simulink model "StartFromStrach"  (Simulink 8.8)
settings: Solver=FixedStepDiscrete  StartTime=0.0  StopTime=CONFIG.SIMULATION_TIME  FixedStep=CONFIG.Ts  RelTol=1e-3  EnableMultiTasking=on
InitFcn:
  | cd(fileparts(which(bdroot)));
  | initStartFromScratch;
undefined symbols (not defined in the file or in its folder): CONFIG, ConstraintsFeetMatrix, gain, reg, ROBOT_DOF, sat, sm, upperBoundFeetConstraints, WBT_robotName
libraries: WBToolboxLibrary x47
settings Model: SuppressorTable=22 serialization::archive 11 0 3 0 0 0 11 0  Creator=marie  LastModifiedBy=marie
settings DataIOCC: LimitDataPoints=off  SaveFormat=Dataset  SignalLoggingSaveFormat=Dataset
settings OptimizationCC: LifeSpan=auto
settings DebuggingCC: UnderspecifiedInitializationDetection=Simplified  MergeDetectMultiDrivingBlocksExec=error  FcnCallInpInsideContextMsg=error  StateNameClashWarn=none  SFUnexpectedBacktrackingDiag=error  SFNoUnconditionalDefaultTransitionDiag=error  SFExecutionAtInitializationDiag=warning
settings HardwareCC: ProdBitPerPointer=64  ProdBitPerSizeT=64  ProdBitPerPtrDiffT=64  ProdLargestAtomicFloat=Float  ProdIntDivRoundTo=Zero  ProdEndianess=LittleEndian  ProdWordSize=64  ProdHWDeviceType=Intel->x86-64 (Windows64)
settings ModelReferenceCC: PropagateSignalLabelsOutOfModel=on
settings GRTTargetCC: TargetLangStandard=C99 (ISO)  GeneratePreprocessorConditionals=Use local settings  CombineOutputUpdateFcns=on  GRTInterface=off
settings ConfigComp: CovMetricSettings=dwe  CovHtmlReporting=off  CovSaveCumulativeToWorkspaceVar=off  CovSaveSingleToWorkspaceVar=off  CovExternalEMLEnable=on

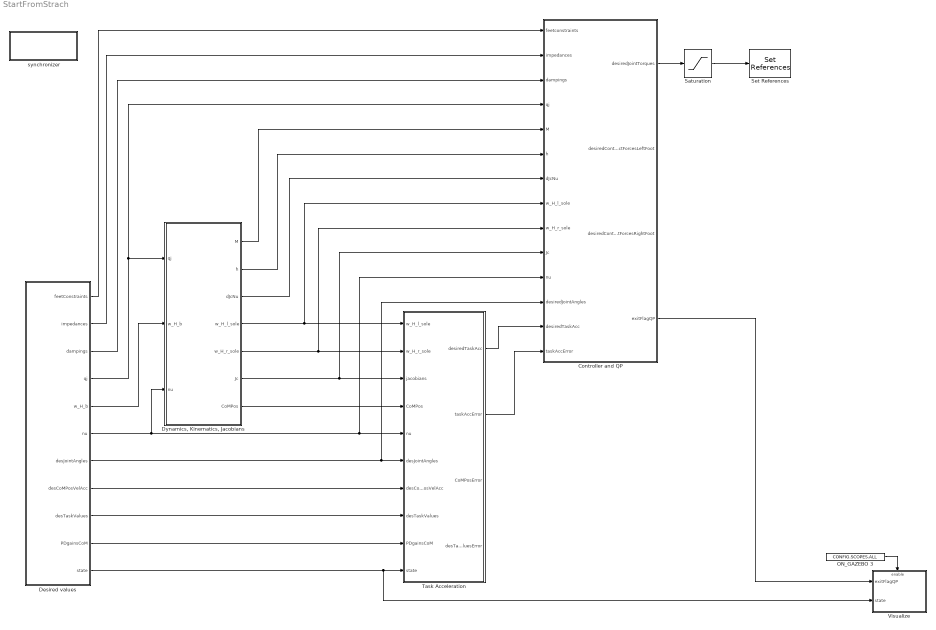
== system StartFromStrach ==
  Controller and QP : Subsystem
  Desired values : Subsystem
  "Dynamics, Kinematics, Jacobians" : Subsystem
  ON_GAZEBO 3 : Constant  Value=CONFIG.SCOPES.ALL
  Saturation : Saturate  UpperLimit=sat.torque  LowerLimit=-sat.torque
  Set References : WBToolboxLibrary/wholeBodyActuators/Set References  controlType=Torque  fullOrSubControl=Full  controlledJoints=''  robotName=WBT_robotName  localName=WBT_modelName  wbiFile=WBT_wbiFilename  wbiList=WBT_wbiList
  Task Acceleration : Subsystem
  Visualize : Subsystem
  synchronizer : Subsystem
      mask Display: disp('SYNCHRONIZER')
  wires:
  Desired values/5(w_H_b) -> "Dynamics, Kinematics, Jacobians"/2(w_H_b)
  Desired values/4(qj) -> "Dynamics, Kinematics, Jacobians"/1(qj), Controller and QP/4(qj)
  "Dynamics, Kinematics, Jacobians"/7(CoMPos) -> Task Acceleration/4(CoMPos)
  Desired values/8(desCoMPosVelAcc) -> Task Acceleration/7(desCoMPosVelAcc)
  Desired values/6(nu) -> Controller and QP/11(nu), Task Acceleration/5(nu), "Dynamics, Kinematics, Jacobians"/3(nu)
  "Dynamics, Kinematics, Jacobians"/6(Jc) -> Controller and QP/10(Jc), Task Acceleration/3(jacobians)
  Desired values/7(desJointAngles) -> Task Acceleration/6(desJointAngles), Controller and QP/12(desiredJointAngles)
  Desired values/9(desTaskValues) -> Task Acceleration/8(desTaskValues)
  Desired values/10(PDgainsCoM) -> Task Acceleration/9(PDgainsCoM)
  "Dynamics, Kinematics, Jacobians"/5(w_H_r_sole) -> Controller and QP/9(w_H_r_sole), Task Acceleration/2(w_H_r_sole)
  "Dynamics, Kinematics, Jacobians"/4(w_H_l_sole) -> Controller and QP/8(w_H_l_sole), Task Acceleration/1(w_H_l_sole)
  Desired values/2(impedances) -> Controller and QP/2(impedances)
  Desired values/1(feetConstraints) -> Controller and QP/1(feetconstraints)
  "Dynamics, Kinematics, Jacobians"/1(M) -> Controller and QP/5(M)
  "Dynamics, Kinematics, Jacobians"/2(h) -> Controller and QP/6(h)
  "Dynamics, Kinematics, Jacobians"/3(dJcNu) -> Controller and QP/7(dJcNu)
  Task Acceleration/1(desiredTaskAcc) -> Controller and QP/13(desiredTaskAcc)
  Task Acceleration/2(taskAccError) -> Controller and QP/14(taskAccError)
  Desired values/3(dampings) -> Controller and QP/3(dampings)
  Controller and QP/1(desiredJointTorques) -> Saturation/1
  Saturation/1 -> Set References/1
  ON_GAZEBO 3/1 -> Visualize/Enable
  Desired values/11(state) -> Visualize/2(state), Task Acceleration/10(state)
  Controller and QP/4(exitFlagQP) -> Visualize/1(exitFlagQP)

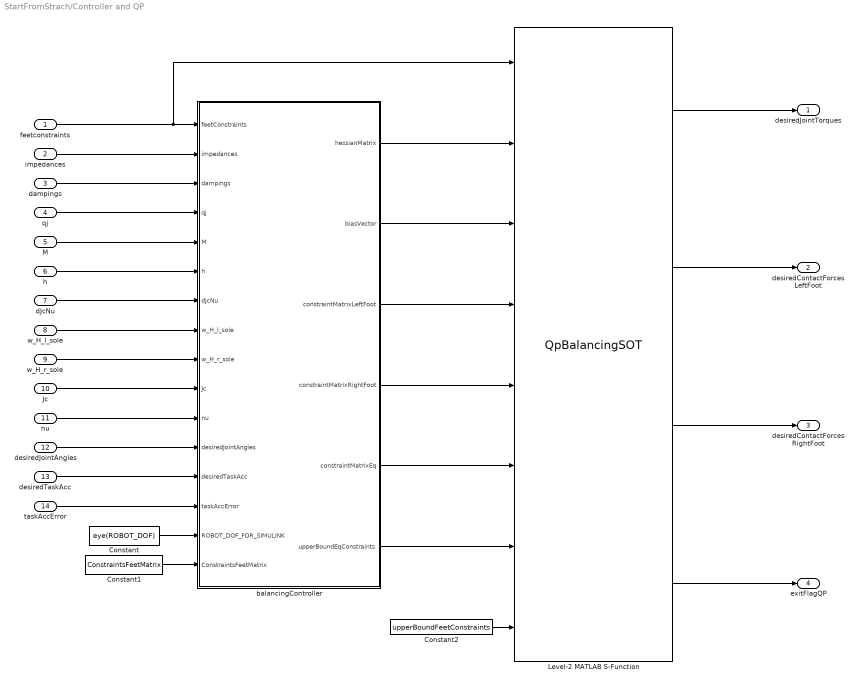
== system StartFromStrach/Controller and QP ==
  feetconstraints : Inport
  impedances : Inport  Port=2
  dampings : Inport  Port=3
  qj : Inport  Port=4
  M : Inport  Port=5
  h : Inport  Port=6
  dJcNu : Inport  Port=7
  w_H_l_sole : Inport  Port=8
  w_H_r_sole : Inport  Port=9
  Jc : Inport  Port=10
  nu : Inport  Port=11
  desiredJointAngles : Inport  Port=12
  desiredTaskAcc : Inport  Port=13
  taskAccError : Inport  Port=14
  Constant : Constant  Value=eye(ROBOT_DOF)
  Constant1 : Constant  Value=ConstraintsFeetMatrix
  Constant2 : Constant  Value=upperBoundFeetConstraints
  Level-2 MATLAB S-Function : M-S-Function  FunctionName=QpBalancingSOT  Parameters=ROBOT_DOF,sat.torqueDot,CONFIG.Ts,CONFIG.QP.USE_CONTINUITY_CONSTRAINTS,CONFIG.QP.USE_STRICT_TASK_PRIORITIES, reg.HessianQP  mask{robotDofs=ROBOT_DOF, tauDotMax=sat.torqueDot, Ts=CONFIG.Ts}
      mask prompts: robotDofs "Robt degrees of freedom"; tauDotMax "Maximum derivative of torques"; Ts "Controller period"
      mask Display: disp('QP')
  balancingController : MATLAB Function  TreatAsAtomicUnit=on
  desiredJointTorques : Outport
  desiredContactForcesLeftFoot : Outport  Port=2
  desiredContactForcesRightFoot : Outport  Port=3
  exitFlagQP : Outport  Port=4
  wires:
  balancingController/1(hessianMatrix) -> Level-2 MATLAB S-Function/2
  feetconstraints/1 -> Level-2 MATLAB S-Function/1, balancingController/1(feetConstraints)
  qj/1 -> balancingController/4(qj)
  impedances/1 -> balancingController/2(impedances)
  M/1 -> balancingController/5(M)
  h/1 -> balancingController/6(h)
  dJcNu/1 -> balancingController/7(dJcNu)
  w_H_l_sole/1 -> balancingController/8(w_H_l_sole)
  w_H_r_sole/1 -> balancingController/9(w_H_r_sole)
  Jc/1 -> balancingController/10(Jc)
  nu/1 -> balancingController/11(nu)
  desiredJointAngles/1 -> balancingController/12(desiredJointAngles)
  desiredTaskAcc/1 -> balancingController/13(desiredTaskAcc)
  taskAccError/1 -> balancingController/14(taskAccError)
  Constant/1 -> balancingController/15(ROBOT_DOF_FOR_SIMULINK)
  Constant1/1 -> balancingController/16(ConstraintsFeetMatrix)
  dampings/1 -> balancingController/3(dampings)
  balancingController/2(biasVector) -> Level-2 MATLAB S-Function/3
  balancingController/3(constraintMatrixLeftFoot) -> Level-2 MATLAB S-Function/4
  balancingController/4(constraintMatrixRightFoot) -> Level-2 MATLAB S-Function/5
  balancingController/5(constraintMatrixEq) -> Level-2 MATLAB S-Function/6
  balancingController/6(upperBoundEqConstraints) -> Level-2 MATLAB S-Function/7
  Constant2/1 -> Level-2 MATLAB S-Function/8
  Level-2 MATLAB S-Function/1 -> desiredJointTorques/1
  Level-2 MATLAB S-Function/2 -> desiredContactForcesLeftFoot/1
  Level-2 MATLAB S-Function/3 -> desiredContactForcesRightFoot/1
  Level-2 MATLAB S-Function/4 -> exitFlagQP/1

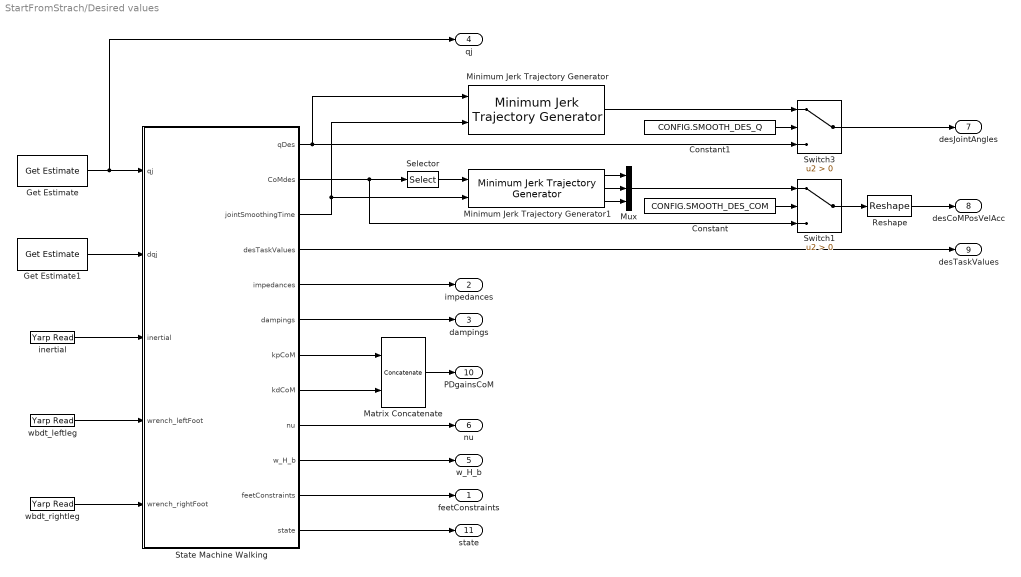
== system StartFromStrach/Desired values ==
  Constant : Constant  Value=CONFIG.SMOOTH_DES_COM
  Constant1 : Constant  Value=CONFIG.SMOOTH_DES_Q
  Get Estimate : WBToolboxLibrary/wholeBodyStates/Get Estimate  estimateType=Joints Position  robotName=WBT_robotName  localName=WBT_modelName  wbiFile=WBT_wbiFilename  wbiList=WBT_wbiList
  Get Estimate1 : WBToolboxLibrary/wholeBodyStates/Get Estimate  estimateType=Joints Velocity  robotName=WBT_robotName  localName=WBT_modelName  wbiFile=WBT_wbiFilename  wbiList=WBT_wbiList
  Matrix Concatenate : Concatenate  Mode=Multidimensional array  ConcatenateDimension=2
  Minimum Jerk Trajectory Generator : WBToolboxLibrary/Utilities/Minimum Jerk Trajectory Generator  externalSettlingTime=on  settlingTime=3  sampleTime=CONFIG.Ts  resetOnSettlingTime=off  firstDerivatives=off  secondDerivatives=off  explicitInitialValue=off
  Minimum Jerk Trajectory Generator1 : WBToolboxLibrary/Utilities/Minimum Jerk Trajectory Generator  externalSettlingTime=on  settlingTime=3  sampleTime=CONFIG.Ts  resetOnSettlingTime=off  firstDerivatives=on  secondDerivatives=on  explicitInitialValue=off
  Mux : Mux  Inputs=3
  Reshape : Reshape  OutputDimensionality=Customize  OutputDimensions=[3,3]
  Selector : Selector  InputPortWidth=9  IndexOptions=Index vector (dialog)  Indices=[1 2 3]  OutputSizes=1
  State Machine Walking : Subsystem
  Switch1 : Switch  Criteria=u2 > Threshold
  Switch3 : Switch  Criteria=u2 > Threshold
  inertial : WBToolboxLibrary/Utilities/Yarp Read  portName=PORTS.IMU  signalSize=12  blocking=off  timestamp=off  autoconnect=on  errorOnConnection=on
  wbdt_leftleg : WBToolboxLibrary/Utilities/Yarp Read  portName=PORTS.WBDT_LEFTLEG_EE  signalSize=6  blocking=off  timestamp=off  autoconnect=on  errorOnConnection=off
  wbdt_rightleg : WBToolboxLibrary/Utilities/Yarp Read  portName=PORTS.WBDT_RIGHTLEG_EE  signalSize=6  blocking=off  timestamp=off  autoconnect=on  errorOnConnection=off
  feetConstraints : Outport
  impedances : Outport  Port=2
  dampings : Outport  Port=3
  qj : Outport  Port=4
  w_H_b : Outport  Port=5
  nu : Outport  Port=6
  desJointAngles : Outport  Port=7
  desCoMPosVelAcc : Outport  Port=8
  desTaskValues : Outport  Port=9
  PDgainsCoM : Outport  Port=10
  state : Outport  Port=11
  wires:
  Minimum Jerk Trajectory Generator/1 -> Switch3/1
  Constant/1 -> Switch1/2
  Constant1/1 -> Switch3/2
  Minimum Jerk Trajectory Generator1/3 -> Mux/3
  Minimum Jerk Trajectory Generator1/2 -> Mux/2
  State Machine Walking/8(kdCoM) -> Matrix Concatenate/2
  Matrix Concatenate/1 -> PDgainsCoM/1
  State Machine Walking/10(w_H_b) -> w_H_b/1
  State Machine Walking/12(state) -> state/1
  Mux/1 -> Switch1/1
  Minimum Jerk Trajectory Generator1/1 -> Mux/1
  State Machine Walking/5(impedances) -> impedances/1
  Selector/1 -> Minimum Jerk Trajectory Generator1/1
  State Machine Walking/3(jointSmoothingTime) -> Minimum Jerk Trajectory Generator/2, Minimum Jerk Trajectory Generator1/2
  Switch1/1 -> Reshape/1
  Switch3/1 -> desJointAngles/1
  State Machine Walking/2(CoMdes) -> Switch1/3, Selector/1
  State Machine Walking/4(desTaskValues) -> desTaskValues/1
  State Machine Walking/11(feetConstraints) -> feetConstraints/1
  State Machine Walking/1(qDes) -> Minimum Jerk Trajectory Generator/1, Switch3/3
  State Machine Walking/9(nu) -> nu/1
  State Machine Walking/7(kpCoM) -> Matrix Concatenate/1
  Reshape/1 -> desCoMPosVelAcc/1
  inertial/1 -> State Machine Walking/3(inertial)
  Get Estimate/1 -> qj/1, State Machine Walking/1(qj)
  Get Estimate1/1 -> State Machine Walking/2(dqj)
  wbdt_leftleg/1 -> State Machine Walking/4(wrench_leftFoot)
  wbdt_rightleg/1 -> State Machine Walking/5(wrench_rightFoot)
  State Machine Walking/6(dampings) -> dampings/1

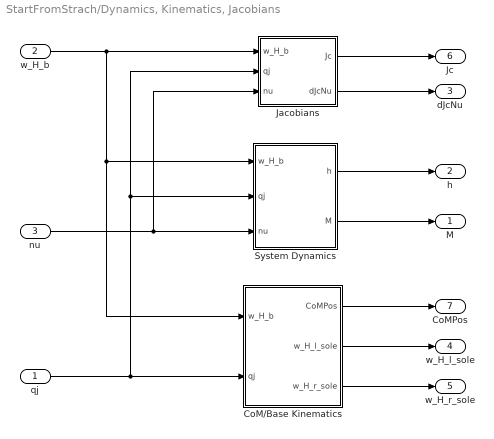
== system StartFromStrach/Dynamics, Kinematics, Jacobians ==
  qj : Inport
  w_H_b : Inport  Port=2
  nu : Inport  Port=3
  CoM/Base Kinematics : Subsystem
  Jacobians : Subsystem
  System Dynamics : Subsystem
  M : Outport
  h : Outport  Port=2
  dJcNu : Outport  Port=3
  w_H_l_sole : Outport  Port=4
  w_H_r_sole : Outport  Port=5
  Jc : Outport  Port=6
  CoMPos : Outport  Port=7
  wires:
  qj/1 -> Jacobians/2(qj), System Dynamics/2(qj), CoM/Base Kinematics/2(qj)
  w_H_b/1 -> CoM/Base Kinematics/1(w_H_b), System Dynamics/1(w_H_b), Jacobians/1(w_H_b)
  CoM/Base Kinematics/1(CoMPos) -> CoMPos/1
  nu/1 -> Jacobians/3(nu), System Dynamics/3(nu)
  Jacobians/1(Jc) -> Jc/1
  Jacobians/2(dJcNu) -> dJcNu/1
  System Dynamics/2(M) -> M/1
  System Dynamics/1(h) -> h/1
  CoM/Base Kinematics/2(w_H_l_sole) -> w_H_l_sole/1
  CoM/Base Kinematics/3(w_H_r_sole) -> w_H_r_sole/1

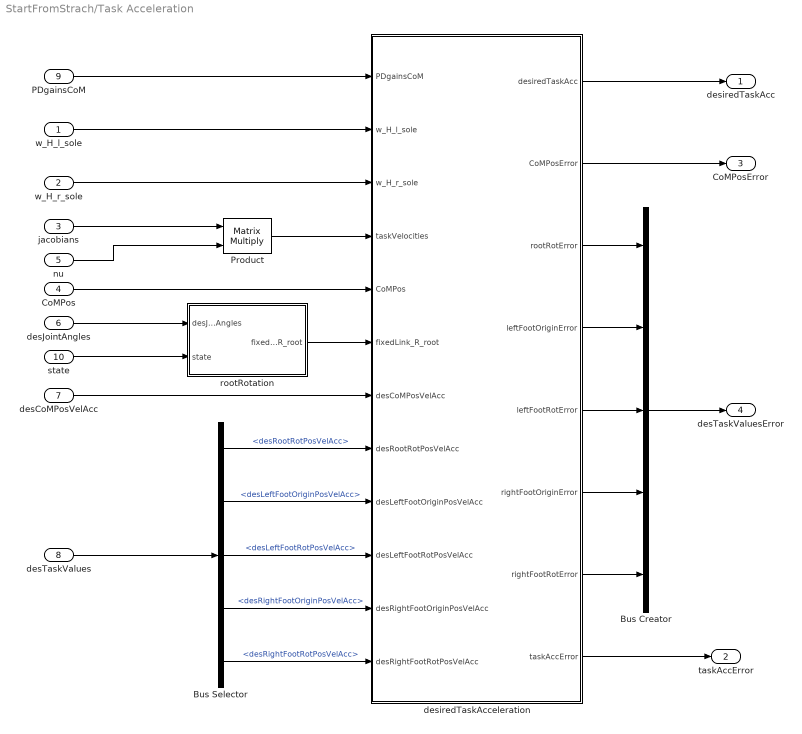
== system StartFromStrach/Task Acceleration ==
  w_H_l_sole : Inport
  w_H_r_sole : Inport  Port=2
  jacobians : Inport  Port=3
  CoMPos : Inport  Port=4
  nu : Inport  Port=5
  desJointAngles : Inport  Port=6
  desCoMPosVelAcc : Inport  Port=7
  desTaskValues : Inport  Port=8
  PDgainsCoM : Inport  Port=9
  state : Inport  Port=10
  Bus Creator : BusCreator  Inputs='rootRotError','leftFootOriginError','leftFootRotError','rightFootOriginError','rightFootRotError'
  Bus Selector : BusSelector  OutputSignals=desRootRotPosVelAcc,desLeftFootOriginPosVelAcc,desLeftFootRotPosVelAcc,desRightFootOriginPosVelAcc,desRightFootRotPosVelAcc
  Product : Product  Multiplication=Matrix(*)
  desiredTaskAcceleration : MATLAB Function  TreatAsAtomicUnit=on
  rootRotation : Subsystem
  desiredTaskAcc : Outport
  taskAccError : Outport  Port=2
  CoMPosError : Outport  Port=3
  desTaskValuesError : Outport  Port=4
  wires:
  state/1 -> rootRotation/2(state)
  Bus Selector/1 -> desiredTaskAcceleration/8(desRootRotPosVelAcc)  "<desRootRotPosVelAcc>"
  Bus Selector/2 -> desiredTaskAcceleration/9(desLeftFootOriginPosVelAcc)  "<desLeftFootOriginPosVelAcc>"
  desJointAngles/1 -> rootRotation/1(desJointAngles)
  Bus Selector/3 -> desiredTaskAcceleration/10(desLeftFootRotPosVelAcc)  "<desLeftFootRotPosVelAcc>"
  Bus Selector/4 -> desiredTaskAcceleration/11(desRightFootOriginPosVelAcc)  "<desRightFootOriginPosVelAcc>"
  desTaskValues/1 -> Bus Selector/1
  rootRotation/1(fixedLink_R_root) -> desiredTaskAcceleration/6(fixedLink_R_root)
  Bus Selector/5 -> desiredTaskAcceleration/12(desRightFootRotPosVelAcc)  "<desRightFootRotPosVelAcc>"
  PDgainsCoM/1 -> desiredTaskAcceleration/1(PDgainsCoM)
  jacobians/1 -> Product/1
  nu/1 -> Product/2
  CoMPos/1 -> desiredTaskAcceleration/5(CoMPos)
  desCoMPosVelAcc/1 -> desiredTaskAcceleration/7(desCoMPosVelAcc)
  Product/1 -> desiredTaskAcceleration/4(taskVelocities)
  desiredTaskAcceleration/3(rootRotError) -> Bus Creator/1
  desiredTaskAcceleration/4(leftFootOriginError) -> Bus Creator/2
  desiredTaskAcceleration/5(leftFootRotError) -> Bus Creator/3
  desiredTaskAcceleration/6(rightFootOriginError) -> Bus Creator/4
  desiredTaskAcceleration/7(rightFootRotError) -> Bus Creator/5
  desiredTaskAcceleration/1(desiredTaskAcc) -> desiredTaskAcc/1
  desiredTaskAcceleration/2(CoMPosError) -> CoMPosError/1
  Bus Creator/1 -> desTaskValuesError/1
  desiredTaskAcceleration/8(taskAccError) -> taskAccError/1
  w_H_r_sole/1 -> desiredTaskAcceleration/3(w_H_r_sole)
  w_H_l_sole/1 -> desiredTaskAcceleration/2(w_H_l_sole)

== system StartFromStrach/Visualize ==
  exitFlagQP : Inport
  state : Inport  Port=2
  Enable : EnablePort
  ON_GAZEBO 4 : Constant  Value=CONFIG.SCOPES.QP
  Visualize eventual QP failures : Subsystem
  wires:
  state/1 -> Visualize eventual QP failures/2(state)
  ON_GAZEBO 4/1 -> Visualize eventual QP failures/Enable
  exitFlagQP/1 -> Visualize eventual QP failures/1(exitFlagQP)

== system StartFromStrach/synchronizer ==
  GAZEBO_SYNCHRONIZER : Subsystem
  Logical Operator : Logic  Operator=NOT  AllPortsSameDT=off  OutDataTypeStr=boolean
  "ON_GAZEBO " : Constant  Value=CONFIG.ON_GAZEBO
  REAL_TIME_SYNC : Subsystem
  wires:
  Logical Operator/1 -> REAL_TIME_SYNC/Enable
  "ON_GAZEBO "/1 -> GAZEBO_SYNCHRONIZER/Enable, Logical Operator/1

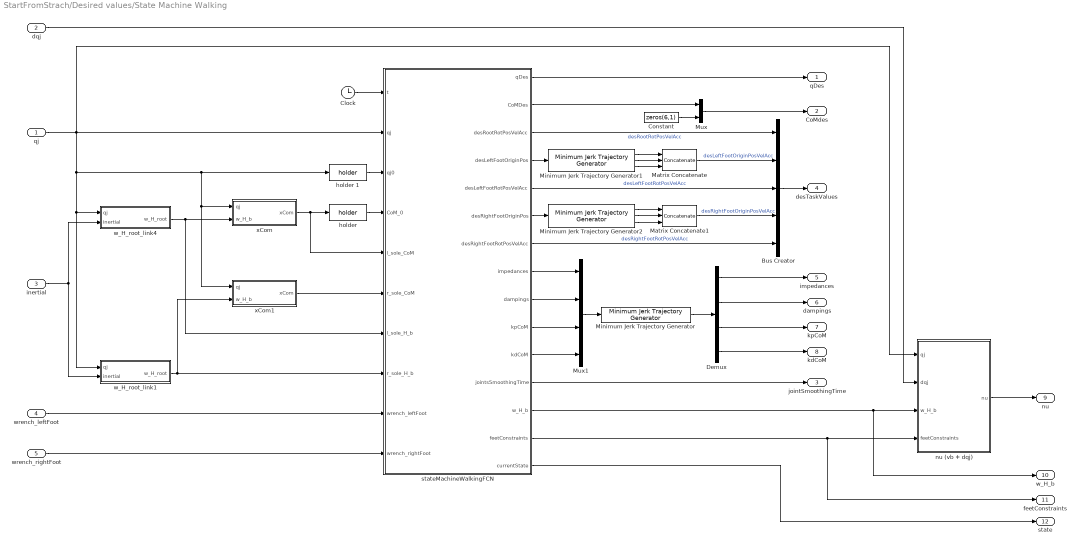
== system StartFromStrach/Desired values/State Machine Walking ==
  qj : Inport
  dqj : Inport  Port=2
  inertial : Inport  Port=3
  wrench_leftFoot : Inport  Port=4
  wrench_rightFoot : Inport  Port=5
  Bus Creator : BusCreator  Inputs='desRootRotPosVelAcc','desLeftFootOriginPosVelAcc','desLeftFootRotPosVelAcc','desRightFootOriginPosVelAcc','desRightFootRotPosVelAcc'
  Clock : Clock
  Constant : Constant  Value=zeros(6,1)
  Demux : Demux  Outputs=[ROBOT_DOF, ROBOT_DOF, 3, 3]
  Matrix Concatenate : Concatenate  NumInputs=3  Mode=Multidimensional array  ConcatenateDimension=2
  Matrix Concatenate1 : Concatenate  NumInputs=3  Mode=Multidimensional array  ConcatenateDimension=2
  Minimum Jerk Trajectory Generator : WBToolboxLibrary/Utilities/Minimum Jerk Trajectory Generator  externalSettlingTime=off  settlingTime=gain.SmoothingTimeGainScheduling  sampleTime=CONFIG.Ts  resetOnSettlingTime=off  firstDerivatives=off  secondDerivatives=off  explicitInitialValue=off
  Minimum Jerk Trajectory Generator1 : WBToolboxLibrary/Utilities/Minimum Jerk Trajectory Generator  externalSettlingTime=off  settlingTime=gain.SmoothingTimeGainScheduling  sampleTime=CONFIG.Ts  resetOnSettlingTime=off  firstDerivatives=on  secondDerivatives=on  explicitInitialValue=off
  Minimum Jerk Trajectory Generator2 : WBToolboxLibrary/Utilities/Minimum Jerk Trajectory Generator  externalSettlingTime=off  settlingTime=gain.SmoothingTimeGainScheduling  sampleTime=CONFIG.Ts  resetOnSettlingTime=off  firstDerivatives=on  secondDerivatives=on  explicitInitialValue=off
  Mux : Mux  Inputs=2
  Mux1 : Mux
  "holder " : WBToolboxLibrary/Utilities/holder 
  holder 1 : WBToolboxLibrary/Utilities/holder 
  nu (vb + dqj) : Subsystem
  stateMachineWalkingFCN : MATLAB Function  TreatAsAtomicUnit=on
  w_H_root_link1 : Subsystem  mask{link_name='r_sole'}
      mask prompts: link_name "link name"
      mask help:
      | This block evaluates the homogeneous transformation between the world and the root link, i.e. ^wH_b. It assumes that the link specified by the variable 'link_name' has a constant position
      | w.r.t. an inertial frame, but it can rotate arbitrarily. This rotation is retrived from the IMU sensor.
      mask Display:
      | str = strrep(link_name, '_','\_');
      | port_label('output',1,['{}^{',str '}H_{root}'],'texmode','on')
      | clear str;
      | 
      | port_label('input',1,'q_j','texmode','on')
      | 
      | port_label('input',2,'inertial','texmode','on')
  w_H_root_link4 : Subsystem  mask{link_name='l_sole'}
      mask prompts: link_name "link name"
      mask help:
      | This block evaluates the homogeneous transformation between the world and the root link, i.e. ^wH_b. It assumes that the link specified by the variable 'link_name' has a constant position
      | w.r.t. an inertial frame, but it can rotate arbitrarily. This rotation is retrived from the IMU sensor.
      mask Display:
      | str = strrep(link_name, '_','\_');
      | port_label('output',1,['{}^{',str '}H_{root}'],'texmode','on')
      | clear str;
      | 
      | port_label('input',1,'q_j','texmode','on')
      | 
      | port_label('input',2,'inertial','texmode','on')
  xCom : Subsystem
  xCom1 : Subsystem
  qDes : Outport
  CoMdes : Outport  Port=2
  jointSmoothingTime : Outport  Port=3
  desTaskValues : Outport  Port=4
  impedances : Outport  Port=5
  dampings : Outport  Port=6
  kpCoM : Outport  Port=7
  kdCoM : Outport  Port=8
  nu : Outport  Port=9
  w_H_b : Outport  Port=10
  feetConstraints : Outport  Port=11
  state : Outport  Port=12
  wires:
  Clock/1 -> stateMachineWalkingFCN/1(t)
  stateMachineWalkingFCN/8(impedances) -> Mux1/1
  stateMachineWalkingFCN/11(kdCoM) -> Mux1/4
  stateMachineWalkingFCN/7(desRightFootRotPosVelAcc) -> Bus Creator/5  "desRightFootRotPosVelAcc"
  Bus Creator/1 -> desTaskValues/1
  wrench_rightFoot/1 -> stateMachineWalkingFCN/10(wrench_rightFoot)
  stateMachineWalkingFCN/10(kpCoM) -> Mux1/3
  stateMachineWalkingFCN/13(w_H_b) -> w_H_b/1, nu (vb + dqj)/3(w_H_b)
  wrench_leftFoot/1 -> stateMachineWalkingFCN/9(wrench_leftFoot)
  Mux1/1 -> Minimum Jerk Trajectory Generator/1
  qj/1 -> nu (vb + dqj)/1(qj), w_H_root_link1/1(qj), w_H_root_link4/1(qj), xCom1/1(qj), xCom/1(qj), holder 1/1, stateMachineWalkingFCN/2(qj)
  nu (vb + dqj)/1(nu) -> nu/1
  holder 1/1 -> stateMachineWalkingFCN/3(qj0)
  xCom1/1(xCom) -> stateMachineWalkingFCN/6(r_sole_CoM)
  "holder "/1 -> stateMachineWalkingFCN/4(CoM_0)
  w_H_root_link4/1(w_H_root) -> stateMachineWalkingFCN/7(l_sole_H_b), xCom/2(w_H_b)
  inertial/1 -> w_H_root_link4/2(inertial), w_H_root_link1/2(inertial)
  xCom/1(xCom) -> "holder "/1, stateMachineWalkingFCN/5(l_sole_CoM)
  Minimum Jerk Trajectory Generator/1 -> Demux/1
  stateMachineWalkingFCN/14(feetConstraints) -> nu (vb + dqj)/4(feetConstraints), feetConstraints/1
  dqj/1 -> nu (vb + dqj)/2(dqj)
  stateMachineWalkingFCN/2(CoMDes) -> Mux/1
  w_H_root_link1/1(w_H_root) -> xCom1/2(w_H_b), stateMachineWalkingFCN/8(r_sole_H_b)
  Demux/1 -> impedances/1
  stateMachineWalkingFCN/12(jointsSmoothingTime) -> jointSmoothingTime/1
  stateMachineWalkingFCN/15(currentState) -> state/1
  stateMachineWalkingFCN/1(qDes) -> qDes/1
  Demux/3 -> kpCoM/1
  Minimum Jerk Trajectory Generator1/1 -> Matrix Concatenate/1
  Minimum Jerk Trajectory Generator1/2 -> Matrix Concatenate/2
  Minimum Jerk Trajectory Generator1/3 -> Matrix Concatenate/3
  Matrix Concatenate/1 -> Bus Creator/2  "desLeftFootOriginPosVelAcc"
  stateMachineWalkingFCN/4(desLeftFootOriginPos) -> Minimum Jerk Trajectory Generator1/1
  Minimum Jerk Trajectory Generator2/1 -> Matrix Concatenate1/1
  Minimum Jerk Trajectory Generator2/2 -> Matrix Concatenate1/2
  Minimum Jerk Trajectory Generator2/3 -> Matrix Concatenate1/3
  stateMachineWalkingFCN/6(desRightFootOriginPos) -> Minimum Jerk Trajectory Generator2/1
  Matrix Concatenate1/1 -> Bus Creator/4  "desRightFootOriginPosVelAcc"
  stateMachineWalkingFCN/3(desRootRotPosVelAcc) -> Bus Creator/1  "desRootRotPosVelAcc"
  stateMachineWalkingFCN/5(desLeftFootRotPosVelAcc) -> Bus Creator/3  "desLeftFootRotPosVelAcc"
  Demux/4 -> kdCoM/1
  Constant/1 -> Mux/2
  Mux/1 -> CoMdes/1
  stateMachineWalkingFCN/9(dampings) -> Mux1/2
  Demux/2 -> dampings/1

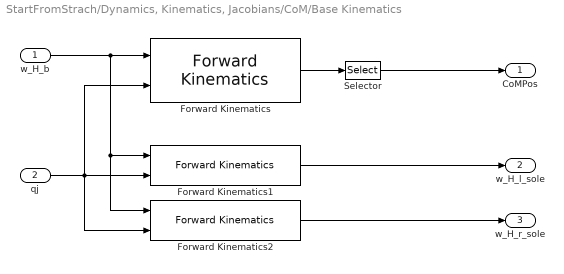
== system StartFromStrach/Dynamics, Kinematics, Jacobians/CoM/Base Kinematics ==
  w_H_b : Inport
  qj : Inport  Port=2
  Forward Kinematics : WBToolboxLibrary/wholeBodyModel/Kinematics/Forward Kinematics  frameName='com'  robotName=WBT_robotName  localName=WBT_modelName  wbiFile=WBT_wbiFilename  wbiList=WBT_wbiList
  Forward Kinematics1 : WBToolboxLibrary/wholeBodyModel/Kinematics/Forward Kinematics  frameName='l_sole'  robotName=WBT_robotName  localName=WBT_modelName  wbiFile=WBT_wbiFilename  wbiList=WBT_wbiList
  Forward Kinematics2 : WBToolboxLibrary/wholeBodyModel/Kinematics/Forward Kinematics  frameName='r_sole'  robotName=WBT_robotName  localName=WBT_modelName  wbiFile=WBT_wbiFilename  wbiList=WBT_wbiList
  Selector : Selector  NumberOfDimensions=2  InputPortWidth=6+ROBOT_DOF  IndexOptions=Index vector (dialog),Index vector (dialog)  Indices=[1:3],[4]  OutputSizes=1,1
  CoMPos : Outport
  w_H_l_sole : Outport  Port=2
  w_H_r_sole : Outport  Port=3
  wires:
  Selector/1 -> CoMPos/1
  qj/1 -> Forward Kinematics1/2, Forward Kinematics2/2, Forward Kinematics/2
  Forward Kinematics/1 -> Selector/1
  w_H_b/1 -> Forward Kinematics1/1, Forward Kinematics2/1, Forward Kinematics/1
  Forward Kinematics2/1 -> w_H_r_sole/1
  Forward Kinematics1/1 -> w_H_l_sole/1

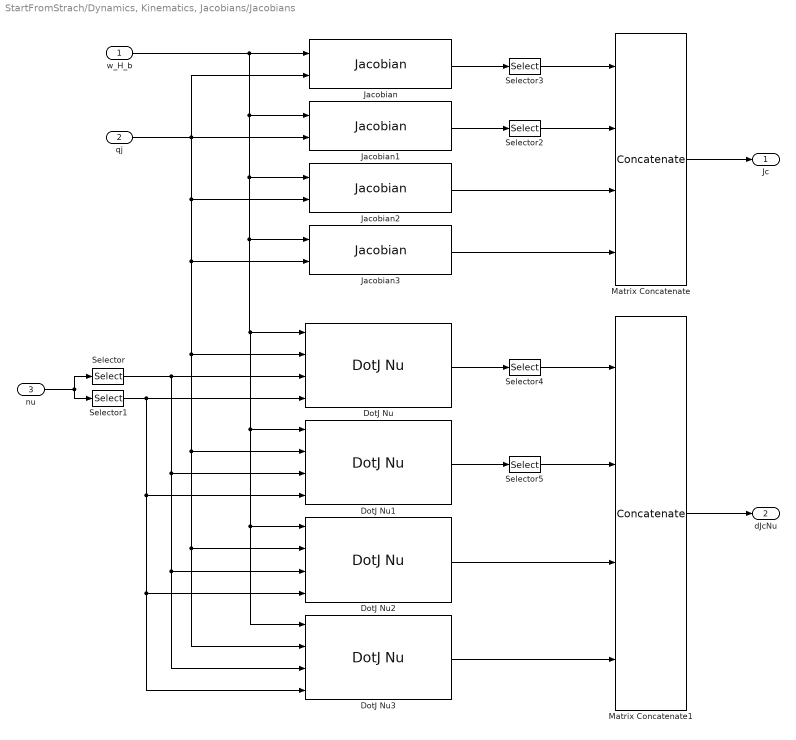
== system StartFromStrach/Dynamics, Kinematics, Jacobians/Jacobians ==
  w_H_b : Inport
  qj : Inport  Port=2
  nu : Inport  Port=3
  DotJ Nu : WBToolboxLibrary/wholeBodyModel/Jacobians/DotJ Nu  frameName='com'  robotName=WBT_robotName  localName=WBT_modelName  wbiFile=WBT_wbiFilename  wbiList=WBT_wbiList
  DotJ Nu1 : WBToolboxLibrary/wholeBodyModel/Jacobians/DotJ Nu  frameName='root_link'  robotName=WBT_robotName  localName=WBT_modelName  wbiFile=WBT_wbiFilename  wbiList=WBT_wbiList
  DotJ Nu2 : WBToolboxLibrary/wholeBodyModel/Jacobians/DotJ Nu  frameName='l_sole'  robotName=WBT_robotName  localName=WBT_modelName  wbiFile=WBT_wbiFilename  wbiList=WBT_wbiList
  DotJ Nu3 : WBToolboxLibrary/wholeBodyModel/Jacobians/DotJ Nu  frameName='r_sole'  robotName=WBT_robotName  localName=WBT_modelName  wbiFile=WBT_wbiFilename  wbiList=WBT_wbiList
  Jacobian : WBToolboxLibrary/wholeBodyModel/Jacobians/Jacobian  frameName='com'  robotName=WBT_robotName  localName=WBT_modelName  wbiFile=WBT_wbiFilename  wbiList=WBT_wbiList
  Jacobian1 : WBToolboxLibrary/wholeBodyModel/Jacobians/Jacobian  frameName='root_link'  robotName=WBT_robotName  localName=WBT_modelName  wbiFile=WBT_wbiFilename  wbiList=WBT_wbiList
  Jacobian2 : WBToolboxLibrary/wholeBodyModel/Jacobians/Jacobian  frameName='l_sole'  robotName=WBT_robotName  localName=WBT_modelName  wbiFile=WBT_wbiFilename  wbiList=WBT_wbiList
  Jacobian3 : WBToolboxLibrary/wholeBodyModel/Jacobians/Jacobian  frameName='r_sole'  robotName=WBT_robotName  localName=WBT_modelName  wbiFile=WBT_wbiFilename  wbiList=WBT_wbiList
  Matrix Concatenate : Concatenate  NumInputs=4  Mode=Multidimensional array
  Matrix Concatenate1 : Concatenate  NumInputs=4  Mode=Multidimensional array
  Selector : Selector  InputPortWidth=6+ROBOT_DOF  IndexOptions=Index vector (dialog)  Indices=[1:6]  OutputSizes=1
  Selector1 : Selector  InputPortWidth=6+ROBOT_DOF  IndexOptions=Index vector (dialog)  Indices=[7:6+ROBOT_DOF]  OutputSizes=1
  Selector2 : Selector  NumberOfDimensions=2  InputPortWidth=6+ROBOT_DOF  IndexOptions=Index vector (dialog),Index vector (dialog)  Indices=[4:6],[1:6+ROBOT_DOF]  OutputSizes=1,1
  Selector3 : Selector  NumberOfDimensions=2  InputPortWidth=6+ROBOT_DOF  IndexOptions=Index vector (dialog),Index vector (dialog)  Indices=[1:3],[1:6+ROBOT_DOF]  OutputSizes=1,1
  Selector4 : Selector  InputPortWidth=6  IndexOptions=Index vector (dialog)  Indices=[1:3]  OutputSizes=1
  Selector5 : Selector  InputPortWidth=6  IndexOptions=Index vector (dialog)  Indices=[4:6]  OutputSizes=1
  Jc : Outport
  dJcNu : Outport  Port=2
  wires:
  w_H_b/1 -> DotJ Nu1/1, DotJ Nu3/1, DotJ Nu2/1, DotJ Nu/1, Jacobian3/1, Jacobian2/1, Jacobian1/1, Jacobian/1
  qj/1 -> DotJ Nu3/2, DotJ Nu2/2, DotJ Nu1/2, DotJ Nu/2, Jacobian3/2, Jacobian2/2, Jacobian/2, Jacobian1/2
  Selector/1 -> DotJ Nu3/3, DotJ Nu2/3, DotJ Nu1/3, DotJ Nu/3
  Selector1/1 -> DotJ Nu1/4, DotJ Nu2/4, DotJ Nu3/4, DotJ Nu/4
  nu/1 -> Selector1/1, Selector/1
  Jacobian/1 -> Selector3/1
  Jacobian1/1 -> Selector2/1
  Selector3/1 -> Matrix Concatenate/1
  Selector2/1 -> Matrix Concatenate/2
  Jacobian2/1 -> Matrix Concatenate/3
  Jacobian3/1 -> Matrix Concatenate/4
  Matrix Concatenate/1 -> Jc/1
  DotJ Nu/1 -> Selector4/1
  DotJ Nu1/1 -> Selector5/1
  Selector4/1 -> Matrix Concatenate1/1
  Selector5/1 -> Matrix Concatenate1/2
  DotJ Nu2/1 -> Matrix Concatenate1/3
  DotJ Nu3/1 -> Matrix Concatenate1/4
  Matrix Concatenate1/1 -> dJcNu/1

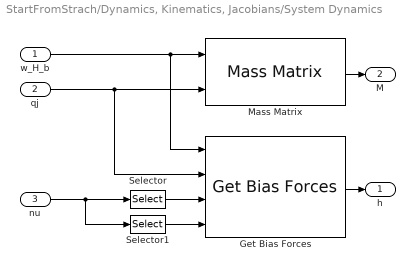
== system StartFromStrach/Dynamics, Kinematics, Jacobians/System Dynamics ==
  w_H_b : Inport
  qj : Inport  Port=2
  nu : Inport  Port=3
  Get Bias Forces : WBToolboxLibrary/wholeBodyModel/Dynamics/Get Bias Forces  robotName=WBT_robotName  localName=WBT_modelName  wbiFile=WBT_wbiFilename  wbiList=WBT_wbiList  explicitGravity=off
  Mass Matrix : WBToolboxLibrary/wholeBodyModel/Dynamics/Mass Matrix  robotName=WBT_robotName  localName=WBT_modelName  wbiFile=WBT_wbiFilename  wbiList=WBT_wbiList
  Selector : Selector  InputPortWidth=6+ROBOT_DOF  IndexOptions=Index vector (dialog)  Indices=[1:6]  OutputSizes=1
  Selector1 : Selector  InputPortWidth=6+ROBOT_DOF  IndexOptions=Index vector (dialog)  Indices=[7:6+ROBOT_DOF]  OutputSizes=1
  h : Outport
  M : Outport  Port=2
  wires:
  Selector/1 -> Get Bias Forces/3
  Selector1/1 -> Get Bias Forces/4
  w_H_b/1 -> Get Bias Forces/1, Mass Matrix/1
  Get Bias Forces/1 -> h/1
  Mass Matrix/1 -> M/1
  qj/1 -> Get Bias Forces/2, Mass Matrix/2
  nu/1 -> Selector1/1, Selector/1

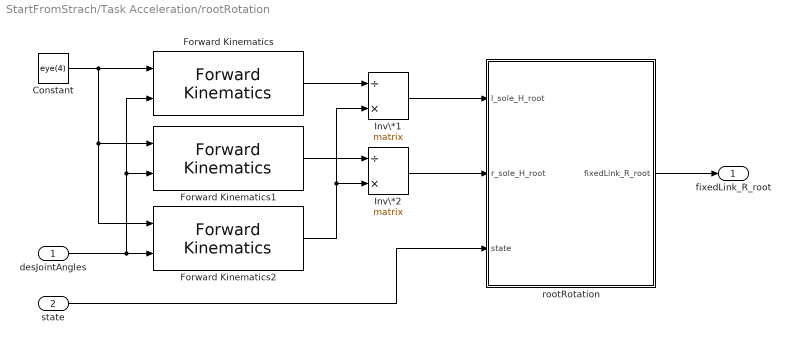
== system StartFromStrach/Task Acceleration/rootRotation ==
  desJointAngles : Inport
  state : Inport  Port=2
  Constant : Constant  Value=eye(4)
  Forward Kinematics : WBToolboxLibrary/wholeBodyModel/Kinematics/Forward Kinematics  frameName='l_sole'  robotName=WBT_robotName  localName=WBT_modelName  wbiFile=WBT_wbiFilename  wbiList=WBT_wbiList
  Forward Kinematics1 : WBToolboxLibrary/wholeBodyModel/Kinematics/Forward Kinematics  frameName='r_sole'  robotName=WBT_robotName  localName=WBT_modelName  wbiFile=WBT_wbiFilename  wbiList=WBT_wbiList
  Forward Kinematics2 : WBToolboxLibrary/wholeBodyModel/Kinematics/Forward Kinematics  frameName='root_link'  robotName=WBT_robotName  localName=WBT_modelName  wbiFile=WBT_wbiFilename  wbiList=WBT_wbiList
  Inv\*1 : Product  Inputs=/*  Multiplication=Matrix(*)
  Inv\*2 : Product  Inputs=/*  Multiplication=Matrix(*)
  rootRotation : MATLAB Function  TreatAsAtomicUnit=on
  fixedLink_R_root : Outport
  wires:
  desJointAngles/1 -> Forward Kinematics/2, Forward Kinematics1/2, Forward Kinematics2/2
  Inv\*2/1 -> rootRotation/2(r_sole_H_root)
  Inv\*1/1 -> rootRotation/1(l_sole_H_root)
  Forward Kinematics2/1 -> Inv\*1/2, Inv\*2/2
  Constant/1 -> Forward Kinematics2/1, Forward Kinematics1/1, Forward Kinematics/1
  Forward Kinematics1/1 -> Inv\*2/1
  Forward Kinematics/1 -> Inv\*1/1
  rootRotation/1(fixedLink_R_root) -> fixedLink_R_root/1
  state/1 -> rootRotation/3(state)

== system StartFromStrach/Visualize/Visualize eventual QP failures ==
  exitFlagQP : Inport
  state : Inport  Port=2
  Enable : EnablePort
  "QP status (0: no failure,  1: not using,  -1 internal error,  -2:  infeasible, -3:  unbounded) " : Scope  NumInputPorts=2
  wires:
  exitFlagQP/1 -> "QP status (0: no failure,  1: not using,  -1 internal error,  -2:  infeasible, -3:  unbounded) "/1  "exitFlagQP"
  state/1 -> "QP status (0: no failure,  1: not using,  -1 internal error,  -2:  infeasible, -3:  unbounded) "/2

== system StartFromStrach/synchronizer/GAZEBO_SYNCHRONIZER ==
  Enable : EnablePort
  Simulator Synchronizer : WBToolboxLibrary/Utilities/Simulator Synchronizer  period=CONFIG.Ts  serverPortName='/clock/rpc'  clientPortName='/WBT_synchronizer/rpc:o'

== system StartFromStrach/synchronizer/REAL_TIME_SYNC ==
  Enable : EnablePort
  Real Time Synchronizer : WBToolboxLibrary/Utilities/Real Time Synchronizer  period=CONFIG.Ts

== system StartFromStrach/Desired values/State Machine Walking/nu (vb + dqj) ==
  qj : Inport
  dqj : Inport  Port=2
  w_H_b : Inport  Port=3
  feetConstraints : Inport  Port=4
  Jacobian : WBToolboxLibrary/wholeBodyModel/Jacobians/Jacobian  frameName='l_sole'  robotName=WBT_robotName  localName=WBT_modelName  wbiFile=WBT_wbiFilename  wbiList=WBT_wbiList
  Jacobian1 : WBToolboxLibrary/wholeBodyModel/Jacobians/Jacobian  frameName='r_sole'  robotName=WBT_robotName  localName=WBT_modelName  wbiFile=WBT_wbiFilename  wbiList=WBT_wbiList
  Mux2 : Mux  Inputs=2
  baseVelocityFCN : MATLAB Function  TreatAsAtomicUnit=on
  nu : Outport
  wires:
  qj/1 -> Jacobian1/2, Jacobian/2
  Jacobian1/1 -> baseVelocityFCN/2(JcRightFoot)
  dqj/1 -> Mux2/2, baseVelocityFCN/4(dqj)
  baseVelocityFCN/1(vb) -> Mux2/1
  w_H_b/1 -> Jacobian/1, Jacobian1/1
  feetConstraints/1 -> baseVelocityFCN/3(feetConstraints)
  Jacobian/1 -> baseVelocityFCN/1(JcLeftFoot)
  Mux2/1 -> nu/1

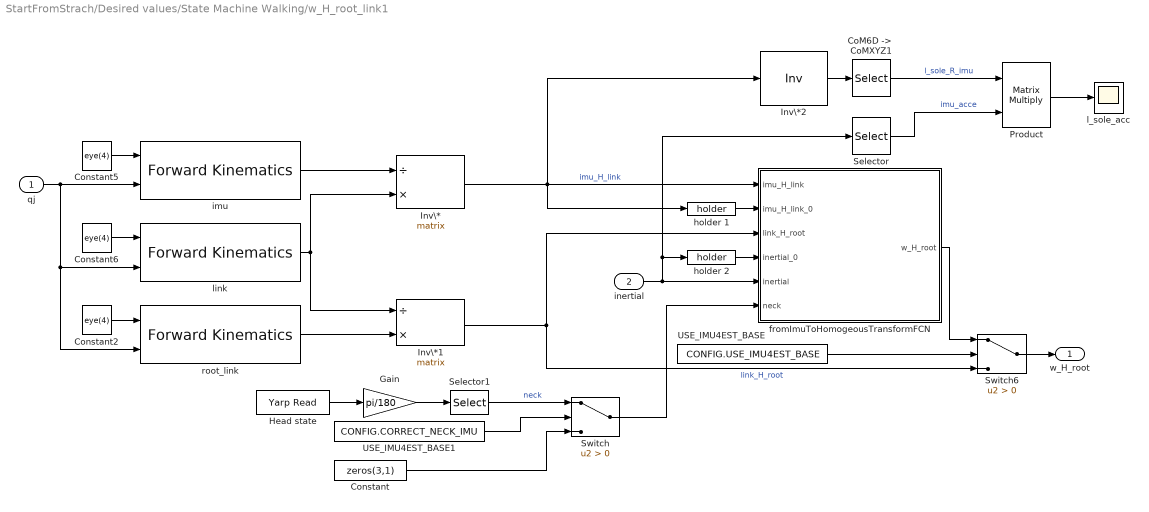
== system StartFromStrach/Desired values/State Machine Walking/w_H_root_link1 ==
  qj : Inport
  inertial : Inport  Port=2
  "CoM6D ->  CoMXYZ1" : Selector  NumberOfDimensions=2  InputPortWidth=7  IndexOptions=Index vector (dialog),Index vector (dialog)  Indices=[1 2 3],[1 2 3]  OutputSizes=1,1
  Constant : Constant  Value=zeros(3,1)
  Constant2 : Constant  Value=eye(4)
  Constant5 : Constant  Value=eye(4)
  Constant6 : Constant  Value=eye(4)
  Gain : Gain  Gain=pi/180
  Head state : WBToolboxLibrary/Utilities/Yarp Read  portName=[WBT_robotName, '/head/state:o']  signalSize=6  blocking=off  timestamp=off  autoconnect=on  errorOnConnection=off
  Inv\* : Product  Inputs=/*  Multiplication=Matrix(*)
  Inv\*1 : Product  Inputs=/*  Multiplication=Matrix(*)
  Inv\*2 : Product  Inputs=/  Multiplication=Matrix(*)
  Product : Product  Multiplication=Matrix(*)
  Selector : Selector  InputPortWidth=12  IndexOptions=Index vector (dialog)  Indices=[4 5 6 ]  OutputSizes=1
  Selector1 : Selector  InputPortWidth=6  IndexOptions=Index vector (dialog)  Indices=[1:3]  OutputSizes=1
  Switch : Switch  Criteria=u2 > Threshold
  Switch6 : Switch  Criteria=u2 > Threshold
  USE_IMU4EST_BASE : Constant  Value=CONFIG.USE_IMU4EST_BASE
  USE_IMU4EST_BASE1 : Constant  Value=CONFIG.CORRECT_NECK_IMU
  fromImuToHomogeousTransformFCN : MATLAB Function  TreatAsAtomicUnit=on
  holder 1 : WBToolboxLibrary/Utilities/holder 
  holder 2 : WBToolboxLibrary/Utilities/holder 
  imu : WBToolboxLibrary/wholeBodyModel/Kinematics/Forward Kinematics  frameName='imu_frame'  robotName=WBT_robotName  localName=WBT_modelName  wbiFile=WBT_wbiFilename  wbiList=WBT_wbiList
  l_sole_acc : Scope
  link : WBToolboxLibrary/wholeBodyModel/Kinematics/Forward Kinematics  frameName=link_name  robotName=WBT_robotName  localName=WBT_modelName  wbiFile=WBT_wbiFilename  wbiList=WBT_wbiList
  root_link : WBToolboxLibrary/wholeBodyModel/Kinematics/Forward Kinematics  frameName='root_link'  robotName=WBT_robotName  localName=WBT_modelName  wbiFile=WBT_wbiFilename  wbiList=WBT_wbiList
  w_H_root : Outport
  wires:
  Constant5/1 -> imu/1
  Inv\*/1 -> Inv\*2/1, holder 1/1, fromImuToHomogeousTransformFCN/1(imu_H_link)  "imu_H_link"
  imu/1 -> Inv\*/1
  Constant6/1 -> link/1
  Inv\*1/1 -> Switch6/3, fromImuToHomogeousTransformFCN/3(link_H_root)  "link_H_root"
  link/1 -> Inv\*/2, Inv\*1/1
  inertial/1 -> Selector/1, holder 2/1, fromImuToHomogeousTransformFCN/5(inertial)
  Switch6/1 -> w_H_root/1
  USE_IMU4EST_BASE/1 -> Switch6/2
  fromImuToHomogeousTransformFCN/1(w_H_root) -> Switch6/1
  Constant2/1 -> root_link/1
  qj/1 -> root_link/2, link/2, imu/2
  root_link/1 -> Inv\*1/2
  holder 1/1 -> fromImuToHomogeousTransformFCN/2(imu_H_link_0)
  holder 2/1 -> fromImuToHomogeousTransformFCN/4(inertial_0)
  Inv\*2/1 -> "CoM6D ->  CoMXYZ1"/1
  "CoM6D ->  CoMXYZ1"/1 -> Product/1  "l_sole_R_imu"
  Selector/1 -> Product/2  "imu_acce"
  Product/1 -> l_sole_acc/1
  Head state/1 -> Gain/1
  Selector1/1 -> Switch/1  "neck"
  USE_IMU4EST_BASE1/1 -> Switch/2
  Switch/1 -> fromImuToHomogeousTransformFCN/6(neck)
  Gain/1 -> Selector1/1
  Constant/1 -> Switch/3

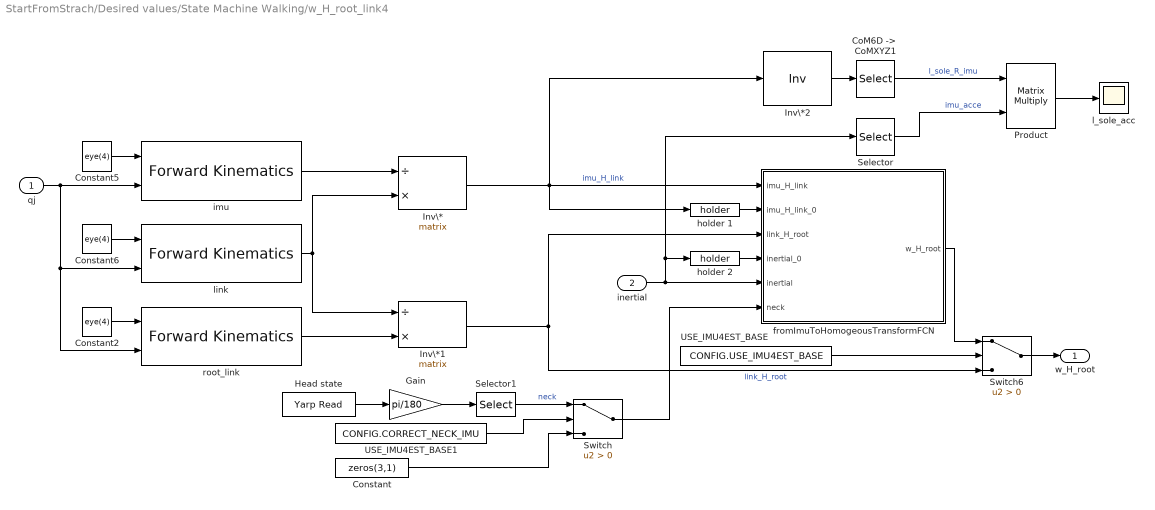
== system StartFromStrach/Desired values/State Machine Walking/w_H_root_link4 ==
  qj : Inport
  inertial : Inport  Port=2
  "CoM6D ->  CoMXYZ1" : Selector  NumberOfDimensions=2  InputPortWidth=7  IndexOptions=Index vector (dialog),Index vector (dialog)  Indices=[1 2 3],[1 2 3]  OutputSizes=1,1
  Constant : Constant  Value=zeros(3,1)
  Constant2 : Constant  Value=eye(4)
  Constant5 : Constant  Value=eye(4)
  Constant6 : Constant  Value=eye(4)
  Gain : Gain  Gain=pi/180
  Head state : WBToolboxLibrary/Utilities/Yarp Read  portName=[WBT_robotName, '/head/state:o']  signalSize=6  blocking=off  timestamp=off  autoconnect=on  errorOnConnection=off
  Inv\* : Product  Inputs=/*  Multiplication=Matrix(*)
  Inv\*1 : Product  Inputs=/*  Multiplication=Matrix(*)
  Inv\*2 : Product  Inputs=/  Multiplication=Matrix(*)
  Product : Product  Multiplication=Matrix(*)
  Selector : Selector  InputPortWidth=12  IndexOptions=Index vector (dialog)  Indices=[4 5 6 ]  OutputSizes=1
  Selector1 : Selector  InputPortWidth=6  IndexOptions=Index vector (dialog)  Indices=[1:3]  OutputSizes=1
  Switch : Switch  Criteria=u2 > Threshold
  Switch6 : Switch  Criteria=u2 > Threshold
  USE_IMU4EST_BASE : Constant  Value=CONFIG.USE_IMU4EST_BASE
  USE_IMU4EST_BASE1 : Constant  Value=CONFIG.CORRECT_NECK_IMU
  fromImuToHomogeousTransformFCN : MATLAB Function  TreatAsAtomicUnit=on
  holder 1 : WBToolboxLibrary/Utilities/holder 
  holder 2 : WBToolboxLibrary/Utilities/holder 
  imu : WBToolboxLibrary/wholeBodyModel/Kinematics/Forward Kinematics  frameName='imu_frame'  robotName=WBT_robotName  localName=WBT_modelName  wbiFile=WBT_wbiFilename  wbiList=WBT_wbiList
  l_sole_acc : Scope
  link : WBToolboxLibrary/wholeBodyModel/Kinematics/Forward Kinematics  frameName=link_name  robotName=WBT_robotName  localName=WBT_modelName  wbiFile=WBT_wbiFilename  wbiList=WBT_wbiList
  root_link : WBToolboxLibrary/wholeBodyModel/Kinematics/Forward Kinematics  frameName='root_link'  robotName=WBT_robotName  localName=WBT_modelName  wbiFile=WBT_wbiFilename  wbiList=WBT_wbiList
  w_H_root : Outport
  wires:
  Constant5/1 -> imu/1
  Inv\*/1 -> Inv\*2/1, holder 1/1, fromImuToHomogeousTransformFCN/1(imu_H_link)  "imu_H_link"
  imu/1 -> Inv\*/1
  Constant6/1 -> link/1
  Inv\*1/1 -> Switch6/3, fromImuToHomogeousTransformFCN/3(link_H_root)  "link_H_root"
  link/1 -> Inv\*/2, Inv\*1/1
  inertial/1 -> Selector/1, holder 2/1, fromImuToHomogeousTransformFCN/5(inertial)
  Switch6/1 -> w_H_root/1
  USE_IMU4EST_BASE/1 -> Switch6/2
  fromImuToHomogeousTransformFCN/1(w_H_root) -> Switch6/1
  Constant2/1 -> root_link/1
  qj/1 -> root_link/2, link/2, imu/2
  root_link/1 -> Inv\*1/2
  holder 1/1 -> fromImuToHomogeousTransformFCN/2(imu_H_link_0)
  holder 2/1 -> fromImuToHomogeousTransformFCN/4(inertial_0)
  Inv\*2/1 -> "CoM6D ->  CoMXYZ1"/1
  "CoM6D ->  CoMXYZ1"/1 -> Product/1  "l_sole_R_imu"
  Selector/1 -> Product/2  "imu_acce"
  Product/1 -> l_sole_acc/1
  Head state/1 -> Gain/1
  Selector1/1 -> Switch/1  "neck"
  USE_IMU4EST_BASE1/1 -> Switch/2
  Switch/1 -> fromImuToHomogeousTransformFCN/6(neck)
  Gain/1 -> Selector1/1
  Constant/1 -> Switch/3

== system StartFromStrach/Desired values/State Machine Walking/xCom ==
  qj : Inport
  w_H_b : Inport  Port=2
  "CoM6D ->  CoMXYZ2" : Selector  NumberOfDimensions=2  InputPortWidth=7  IndexOptions=Index vector (dialog),Index vector (dialog)  Indices=[1 2 3],[4]  OutputSizes=1,1
  com : WBToolboxLibrary/wholeBodyModel/Kinematics/Forward Kinematics  frameName='com'  robotName=WBT_robotName  localName=WBT_modelName  wbiFile=WBT_wbiFilename  wbiList=WBT_wbiList
  xCom : Outport
  wires:
  qj/1 -> com/2
  "CoM6D ->  CoMXYZ2"/1 -> xCom/1
  com/1 -> "CoM6D ->  CoMXYZ2"/1
  w_H_b/1 -> com/1

== system StartFromStrach/Desired values/State Machine Walking/xCom1 ==
  qj : Inport
  w_H_b : Inport  Port=2
  "CoM6D ->  CoMXYZ2" : Selector  NumberOfDimensions=2  InputPortWidth=7  IndexOptions=Index vector (dialog),Index vector (dialog)  Indices=[1 2 3],[4]  OutputSizes=1,1
  com : WBToolboxLibrary/wholeBodyModel/Kinematics/Forward Kinematics  frameName='com'  robotName=WBT_robotName  localName=WBT_modelName  wbiFile=WBT_wbiFilename  wbiList=WBT_wbiList
  xCom : Outport
  wires:
  w_H_b/1 -> com/1
  com/1 -> "CoM6D ->  CoMXYZ2"/1
  "CoM6D ->  CoMXYZ2"/1 -> xCom/1
  qj/1 -> com/2

== matlab function Desired values/State Machine Walking/nu (vb + dqj)/baseVelocityFCN ==
  data: JcLeftFoot input double; vb output double; JcRightFoot input double; feetConstraints input double; dqj input double; reg parameter double
function vb = baseVelocityFCN(JcLeftFoot, JcRightFoot, feetConstraints, dqj, reg)

vb = baseVelocity(JcLeftFoot, JcRightFoot, feetConstraints, dqj, reg);

== matlab function Desired values/State Machine Walking/stateMachineWalkingFCN ==
  data: t input double; qDes output double; qj input double; qj0 input double; CoM_0 input double; l_sole_CoM input double; r_sole_CoM input double; l_sole_H_b input double; r_sole_H_b input double; wrench_leftFoot input double; wrench_rightFoot input double; CoMDes output double; desRootRotPosVelAcc output double; desLeftFootOriginPos output double; desLeftFootRotPosVelAcc output double; desRightFootOriginPos output double; desRightFootRotPosVelAcc output double; impedances output double; dampings output double; kpCoM output double; kdCoM output double; jointsSmoothingTime output double; w_H_b output double; feetConstraints output double; currentState output double; sm parameter double; gain parameter double
function [qDes, CoMDes, desRootRotPosVelAcc, ...
    desLeftFootOriginPos, desLeftFootRotPosVelAcc, desRightFootOriginPos, desRightFootRotPosVelAcc,  ...
    impedances, dampings, kpCoM, kdCoM, jointsSmoothingTime, w_H_b, feetConstraints, currentState] ...
    = stateMachineWalkingFCN(t, qj, qj0, CoM_0, ...
    l_sole_CoM, r_sole_CoM, l_sole_H_b, r_sole_H_b, ...
    wrench_leftFoot, wrench_rightFoot, sm, gain)

[w_H_b, CoMDes, qDes,feetConstraints, impedances, dampings, kpCoM, kdCoM, currentState, jointsSmoothingTime,...
          desRootRotPosVelAcc, desLeftFootRotPosVelAcc, desLeftFootOriginPos, desRightFootRotPosVelAcc, desRightFootOriginPos] = ...
    stateMachineWalking(CoM_0, qj0, l_sole_CoM,r_sole_CoM, qj, t,...
        wrench_rightFoot, wrench_leftFoot, l_sole_H_b, r_sole_H_b, sm, gain);

== matlab function Task Acceleration/rootRotation/rootRotation ==
  data: l_sole_H_root input double; fixedLink_R_root output double; r_sole_H_root input double; state input double
function fixedLink_R_root = rootRotationFCN(l_sole_H_root, r_sole_H_root, state)

fixedLink_R_root = rootRotation(l_sole_H_root, r_sole_H_root, state);

== matlab function Task Acceleration/desiredTaskAcceleration ==
  data: PDgainsCoM input double; desiredTaskAcc output double; w_H_l_sole input double; w_H_r_sole input double; taskVelocities input double; CoMPos input double; fixedLink_R_root input double; desCoMPosVelAcc input double; desRootRotPosVelAcc input double; desLeftFootOriginPosVelAcc input double; desLeftFootRotPosVelAcc input double; desRightFootOriginPosVelAcc input double; desRightFootRotPosVelAcc input double; CoMPosError output double; rootRotError output double; leftFootOriginError output double; leftFootRotError output double; rightFootOriginError output double; rightFootRotError output double; taskAccError output double; gain parameter double
function [desiredTaskAcc, CoMPosError, rootRotError, leftFootOriginError, leftFootRotError, rightFootOriginError, rightFootRotError, taskAccError] = ...
    desiredTaskAccelerationFCN(PDgainsCoM, ...
    w_H_l_sole, w_H_r_sole, taskVelocities, CoMPos, fixedLink_R_root,...
    desCoMPosVelAcc, desRootRotPosVelAcc,...
    desLeftFootOriginPosVelAcc,  desLeftFootRotPosVelAcc, ...
    desRightFootOriginPosVelAcc, desRightFootRotPosVelAcc, gain)

 [desiredTaskAcc,CoMPosError,rootRotError,leftFootOriginError,leftFootRotError,rightFootOriginError,rightFootRotError, taskAccError] = ...
              desiredTaskAcceleration(CoMPos,desCoMPosVelAcc,...
                                      fixedLink_R_root,desRootRotPosVelAcc,...
                                      w_H_l_sole,desLeftFootRotPosVelAcc,desLeftFootOriginPosVelAcc,...
                                      w_H_r_sole,desRightFootRotPosVelAcc,desRightFootOriginPosVelAcc,...
                                      taskVelocities,PDgainsCoM,gain);

== matlab function Controller and QP/balancingController ==
  data: feetConstraints input double; hessianMatrix output double; impedances input double; dampings input double; qj input double; M input double; h input double; dJcNu input double; w_H_l_sole input double; w_H_r_sole input double; Jc input double; nu input double; desiredJointAngles input double; desiredTaskAcc input double; taskAccError input double; biasVector output double; constraintMatrixLeftFoot output double; constraintMatrixRightFoot output double; constraintMatrixEq output double; upperBoundEqConstraints output double; ROBOT_DOF_FOR_SIMULINK input double; ConstraintsFeetMatrix input double; gain parameter double; CONFIG parameter double; reg parameter double
function [hessianMatrix, biasVector, ...
          constraintMatrixLeftFoot, constraintMatrixRightFoot, ...
          constraintMatrixEq, upperBoundEqConstraints] = ...
          balancingControllerSOT_FCN(feetConstraints, impedances, dampings, qj, ...
                                     M, h, dJcNu, w_H_l_sole, w_H_r_sole, Jc, nu, ...
                                     desiredJointAngles, desiredTaskAcc, taskAccError, ...
                                     ROBOT_DOF_FOR_SIMULINK, ConstraintsFeetMatrix, ...
                                     gain, CONFIG, reg)

[hessianMatrix,biasVector,constraintMatrixLeftFoot,constraintMatrixRightFoot,constraintMatrixEq, upperBoundEqConstraints] = ...
                                        balancingControllerSOT(feetConstraints,ROBOT_DOF_FOR_SIMULINK,ConstraintsFeetMatrix,...
                                                               qj,desiredJointAngles, M, h, ...
                                                               Jc, dJcNu, nu,...
                                                               w_H_l_sole, w_H_r_sole, desiredTaskAcc, taskAccError, ...
                                                               impedances, dampings, ...
                                                               gain, CONFIG, reg);

== matlab function Desired values/State Machine Walking/w_H_root_link1/fromImuToHomogeousTransformFCN ==
  data: imu_H_link input double; imu_H_link_0 input double; link_H_root input double; inertial_0 input double; inertial input double; neck input double; w_H_root output double; CONFIG parameter double
function w_H_root = fromBaseToWorldWithImuFCN(imu_H_link,imu_H_link_0,link_H_root,inertial_0,inertial,neck,CONFIG)
%#codegen
w_H_root = fromBaseToWorldWithImu(imu_H_link,imu_H_link_0,link_H_root,inertial_0,inertial,neck,CONFIG);

== matlab function Desired values/State Machine Walking/w_H_root_link4/fromImuToHomogeousTransformFCN ==
  data: imu_H_link input double; imu_H_link_0 input double; link_H_root input double; inertial_0 input double; inertial input double; neck input double; w_H_root output double; CONFIG parameter double
function w_H_root = fromBaseToWorldWithImuFCN(imu_H_link,imu_H_link_0,link_H_root,inertial_0,inertial,neck,CONFIG)
%#codegen
w_H_root = fromBaseToWorldWithImu(imu_H_link,imu_H_link_0,link_H_root,inertial_0,inertial,neck,CONFIG);
